simulink model "sampleModel1942"  (R2023a)
settings: Solver=VariableStepAuto  StartTime=0.0  StopTime=10.0  RelTol=1e-3
libraries: hdlsllib x5
settings Model: Creator=user1  LastModifiedBy=user1

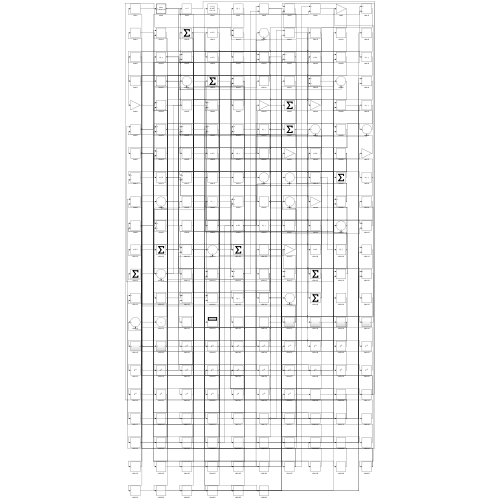
[thumbnail: Simulink's stored preview of the top-level diagram]
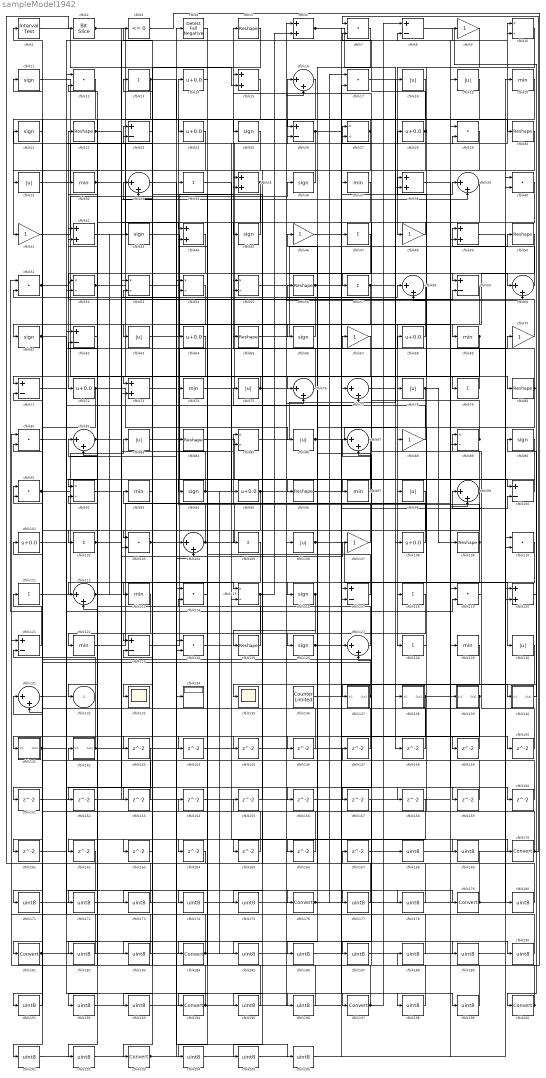
== system sampleModel1942 ==
  cfblk1 : hdlsllib/Logic and Bit Operations/Interval Test  IntervalClosedRight=on  uplimit=0.5  IntervalClosedLeft=on  lowlimit=-0.5  OutDataTypeStr=boolean
  cfblk{10,27,52..55,85,89,92,115} (10 alike) : Product  Inputs=*/  RndMeth=Zero  SaturateOnIntegerOverflow=on
  cfblk{8,23,26,59,62,71,100,117,121,123} (10 alike) : Sum  Inputs=+-
  cfblk{14,24,28,64,68,72,95,101,108} (9 alike) : Bias  Bias=0.0  SaturateOnIntegerOverflow=off
  cfblk{13,34,47,57,79,102,105,111,118,128} (10 alike) : Sum  Inputs=+
  cfblk{7,12,17,29,40,51,81,91,103,110,114,119,124} (13 alike) : DotProduct  OutDataTypeStr=Inherit: Inherit via internal rule
  cfblk{16,33,39,58,60,76..77,82,87,99,104,112,127,131} (14 alike) : Sum  Inputs=|++
  cfblk{18..19,31,63,75,78,83,86,98,106,130} (11 alike) : Abs  SaturateOnIntegerOverflow=off
  cfblk{9,41,46,48,67,70,88,107} (8 alike) : Gain
  cfblk{5,22,30,50,56,65,80,84,96,109,125} (11 alike) : Reshape
  cfblk{11,21,25,36,43,45,61,66,90,94,116,126} (12 alike) : Signum
  cfblk{20,32,37,69,74,93,97,113,122,129} (10 alike) : MinMax
  cfblk{6,15,35,38,42,44,49,73,120} (9 alike) : Sum
  cfblk133 : Scope
  cfblk134 : Display
  cfblk135 : Scope
  cfblk136 : hdlsllib/Sources/Counter Limited  uplimit=7  tsamp=-1
  cfblk137 : Subsystem
      settings: LibrarySourceBlock=|
      | hdlsllib/Ports &
      | Subsystems/Subsystem
  cfblk138 : Subsystem
      settings: LibrarySourceBlock=|
      | hdlsllib/Ports &
      | Subsystems/Subsystem
  cfblk139 : Subsystem
      settings: LibrarySourceBlock=|
      | hdlsllib/Ports &
      | Subsystems/Subsystem
  cfblk140 : Subsystem
      settings: LibrarySourceBlock=|
      | hdlsllib/Ports &
      | Subsystems/Subsystem
  cfblk141 : Subsystem
      settings: LibrarySourceBlock=|
      | hdlsllib/Ports &
      | Subsystems/Subsystem
  cfblk142 : Subsystem
      settings: LibrarySourceBlock=|
      | hdlsllib/Ports &
      | Subsystems/Subsystem
  cfblk{143..167} (25 alike) : Delay  SampleTime=1
  cfblk{168..169,171..175,177..178,180,182..183,185..193,195..196,198..199,201..202,204..206} (30 alike) : DataTypeConversion  OutDataTypeStr=uint8  SaturateOnIntegerOverflow=off  RndMeth=Floor
  cfblk{170,176,179,181,184,194,197,200,203} (9 alike) : DataTypeConversion  SaturateOnIntegerOverflow=off  RndMeth=Floor
  cfblk2 : hdlsllib/Logic and Bit Operations/Bit Slice  lidx=7  ridx=0
  cfblk3 : hdlsllib/Logic and Bit Operations/Compare To Zero  relop=<=  OutDataTypeStr=boolean
  cfblk4 : hdlsllib/Logic and Bit Operations/Detect Fall Negative  vinit=0  OutDataTypeStr=boolean
  cfblk132 : Outport  VectorParamsAs1DForOutWhenUnconnected=off
  wires:
  cfblk111/1 -> cfblk83/1
  cfblk19/1 -> cfblk41/1
  cfblk6/1 -> cfblk108/1, cfblk150/1
  cfblk76/1 -> cfblk5/1
  cfblk126/1 -> cfblk127/1, cfblk169/1
  cfblk2/1 -> cfblk76/1, cfblk30/1
  cfblk124/1 -> cfblk170/1
  cfblk45/1 -> cfblk21/1
  cfblk117/1 -> cfblk93/1
  cfblk78/1 -> cfblk109/1, cfblk146/1
  cfblk15/1 -> cfblk25/1
  cfblk37/1 -> cfblk203/1
  cfblk44/1 -> cfblk72/1
  cfblk43/1 -> cfblk100/1
  cfblk58/1 -> cfblk128/1
  cfblk122/1 -> cfblk85/1
  cfblk114/1 -> cfblk194/1
  cfblk8/1 -> cfblk137/1(In1)
  cfblk33/1 -> cfblk176/1
  cfblk123/1 -> cfblk68/1
  cfblk7/1 -> cfblk126/1
  cfblk66/1 -> cfblk11/1
  cfblk116/1 -> cfblk125/1, cfblk165/1
  cfblk74/1 -> cfblk27/1
  cfblk28/1 -> cfblk116/1, cfblk38/2, cfblk7/2
  cfblk5/1 -> cfblk103/1
  cfblk93/1 -> cfblk23/1
  cfblk42/1 -> cfblk16/1
  cfblk41/1 -> cfblk36/1
  cfblk98/1 -> cfblk113/1
  cfblk138/1(Out1) -> cfblk70/1, cfblk152/1
  cfblk25/1 -> cfblk132/1
  cfblk71/1 -> cfblk67/1
  cfblk115/1 -> cfblk6/2, cfblk193/1
  cfblk139/1(Out1) -> cfblk51/1, cfblk191/1
  cfblk52/1 -> cfblk102/1, cfblk59/2
  cfblk109/1 -> cfblk14/1, cfblk145/1
  cfblk105/1 -> cfblk112/1
  cfblk11/1 -> cfblk99/2
  cfblk99/1 -> cfblk15/1, cfblk175/1
  cfblk107/1 -> cfblk3/1
  cfblk10/1 -> cfblk48/1
  cfblk60/1 -> cfblk49/1
  cfblk84/1 -> cfblk96/1
  cfblk106/1 -> cfblk130/1, cfblk149/1
  cfblk20/1 -> cfblk184/1
  cfblk65/1 -> cfblk19/1
  cfblk85/1 -> cfblk18/1
  cfblk26/1 -> cfblk61/1, cfblk185/1, cfblk190/1
  cfblk86/1 -> cfblk88/1, cfblk39/1, cfblk140/1(In1)
  cfblk61/1 -> cfblk98/1, cfblk159/1, cfblk177/1
  cfblk112/1 -> cfblk107/1, cfblk43/1
  cfblk120/1 -> cfblk200/1
  cfblk36/1 -> cfblk31/1
  cfblk82/1 -> cfblk115/1, cfblk39/2
  cfblk89/1 -> cfblk65/1, cfblk53/2
  cfblk48/1 -> cfblk45/1
  cfblk27/1 -> cfblk24/1, cfblk112/2
  cfblk137/1(Out1) -> cfblk1/1, cfblk71/2
  cfblk21/1 -> cfblk71/1
  cfblk56/1 -> cfblk158/1, cfblk198/1
  cfblk23/1 -> cfblk123/1
  cfblk104/1 -> cfblk74/1, cfblk10/2
  cfblk63/1 -> cfblk35/1
  cfblk140/1(Out1) -> cfblk90/1
  cfblk92/1 -> cfblk85/2
  cfblk70/1 -> cfblk22/1
  cfblk1/1 -> cfblk15/2
  cfblk97/1 -> cfblk56/1
  cfblk17/1 -> cfblk59/1
  cfblk59/1 -> cfblk133/1
  cfblk75/1 -> cfblk55/1, cfblk73/1, cfblk79/1
  cfblk29/1 -> cfblk141/1(In1)
  cfblk127/1 -> cfblk34/1
  cfblk9/1 -> cfblk78/1
  cfblk128/1 -> cfblk38/1
  cfblk100/1 -> cfblk97/1
  cfblk142/1(Out1) -> cfblk17/2, cfblk91/1
  cfblk102/1 -> cfblk9/1, cfblk54/2
  cfblk68/1 -> cfblk66/1
  cfblk4/1 -> cfblk94/1
  cfblk72/1 -> cfblk134/1, cfblk86/1, cfblk201/1
  cfblk55/1 -> cfblk60/1
  cfblk31/1 -> cfblk10/1
  cfblk51/1 -> cfblk52/1, cfblk8/2
  cfblk101/1 -> cfblk28/1
  cfblk39/1 -> cfblk57/1
  cfblk125/1 -> cfblk32/1
  cfblk141/1(Out1) -> cfblk62/1, cfblk77/2, cfblk119/2
  cfblk32/1 -> cfblk44/1, cfblk26/2
  cfblk79/1 -> cfblk27/2
  cfblk69/1 -> cfblk135/1, cfblk127/2
  cfblk88/1 -> cfblk75/1
  cfblk12/1 -> cfblk181/1
  cfblk50/1 -> cfblk69/1
  cfblk113/1 -> cfblk122/1
  cfblk108/1 -> cfblk64/1
  cfblk13/1 -> cfblk63/1, cfblk26/1, cfblk162/1
  cfblk95/1 -> cfblk58/1, cfblk60/2, cfblk161/1
  cfblk46/1 -> cfblk179/1
  cfblk35/1 -> cfblk82/2, cfblk105/1
  cfblk62/1 -> cfblk42/1
  cfblk103/1 -> cfblk50/1, cfblk206/1
  cfblk83/1 -> cfblk115/2
  cfblk136/1 -> cfblk100/2
  cfblk57/1 -> cfblk138/1(In1), cfblk73/2
  cfblk53/1 -> cfblk139/1(In1)
  cfblk80/1 -> cfblk118/1, cfblk55/2
  cfblk121/1 -> cfblk111/1
  cfblk91/1 -> cfblk4/1, cfblk196/1
  cfblk67/1 -> cfblk92/1
  cfblk22/1 -> cfblk80/1, cfblk156/1
  cfblk94/1 -> cfblk29/2, cfblk84/1
  cfblk81/1 -> cfblk197/1
  cfblk119/1 -> cfblk89/1
  cfblk18/1 -> cfblk143/1
  cfblk14/1 -> cfblk144/1
  cfblk145/1 -> cfblk16/2
  cfblk146/1 -> cfblk53/1
  cfblk147/1 -> cfblk23/2
  cfblk77/1 -> cfblk148/1
  cfblk148/1 -> cfblk82/1
  cfblk149/1 -> cfblk54/1
  cfblk150/1 -> cfblk99/1
  cfblk64/1 -> cfblk151/1
  cfblk151/1 -> cfblk76/2
  cfblk152/1 -> cfblk103/2
  cfblk118/1 -> cfblk153/1
  cfblk153/1 -> cfblk62/2
  cfblk154/1 -> cfblk29/1
  cfblk155/1 -> cfblk35/2
  cfblk156/1 -> cfblk89/2
  cfblk110/1 -> cfblk157/1
  cfblk159/1 -> cfblk44/2
  cfblk38/1 -> cfblk160/1
  cfblk160/1 -> cfblk51/2
  cfblk161/1 -> cfblk52/2
  cfblk24/1 -> cfblk163/1
  cfblk163/1 -> cfblk123/2
  cfblk90/1 -> cfblk164/1
  cfblk164/1 -> cfblk2/1
  cfblk165/1 -> cfblk91/2
  cfblk34/1 -> cfblk166/1
  cfblk166/1 -> cfblk42/2
  cfblk167/1 -> cfblk168/1
  cfblk168/1 -> cfblk7/1
  cfblk169/1 -> cfblk167/1
  cfblk170/1 -> cfblk58/2, cfblk101/1
  cfblk54/1 -> cfblk171/1
  cfblk171/1 -> cfblk124/1
  cfblk162/1 -> cfblk172/1
  cfblk172/1 -> cfblk124/2
  cfblk40/1 -> cfblk173/1
  cfblk173/1 -> cfblk142/1(In1)
  cfblk144/1 -> cfblk174/1
  cfblk174/1 -> cfblk40/1
  cfblk175/1 -> cfblk40/2
  cfblk176/1 -> cfblk49/2, cfblk17/1
  cfblk177/1 -> cfblk33/1
  cfblk96/1 -> cfblk178/1
  cfblk178/1 -> cfblk33/2
  cfblk179/1 -> cfblk155/1, cfblk154/1
  cfblk49/1 -> cfblk180/1
  cfblk180/1 -> cfblk46/1
  cfblk181/1 -> cfblk104/2, cfblk119/1
  cfblk143/1 -> cfblk182/1
  cfblk182/1 -> cfblk12/1
  cfblk16/1 -> cfblk183/1
  cfblk183/1 -> cfblk12/2
  cfblk184/1 -> cfblk121/1, cfblk95/1
  cfblk185/1 -> cfblk20/1
  cfblk87/1 -> cfblk186/1
  cfblk186/1 -> cfblk110/1
  cfblk157/1 -> cfblk187/1
  cfblk187/1 -> cfblk87/1
  cfblk3/1 -> cfblk188/1
  cfblk188/1 -> cfblk87/2
  cfblk131/1 -> cfblk189/1
  cfblk189/1 -> cfblk110/2
  cfblk190/1 -> cfblk131/1
  cfblk191/1 -> cfblk131/2
  cfblk47/1 -> cfblk192/1
  cfblk192/1 -> cfblk106/1
  cfblk193/1 -> cfblk47/1
  cfblk194/1 -> cfblk92/2, cfblk77/1
  cfblk130/1 -> cfblk195/1
  cfblk195/1 -> cfblk114/1
  cfblk196/1 -> cfblk114/2
  cfblk197/1 -> cfblk121/2, cfblk6/1, cfblk8/1
  cfblk198/1 -> cfblk81/1
  cfblk73/1 -> cfblk199/1
  cfblk199/1 -> cfblk81/2
  cfblk200/1 -> cfblk147/1, cfblk13/1
  cfblk201/1 -> cfblk120/1
  cfblk158/1 -> cfblk202/1
  cfblk202/1 -> cfblk120/2
  cfblk203/1 -> cfblk104/1, cfblk117/1
  cfblk30/1 -> cfblk204/1
  cfblk204/1 -> cfblk37/1
  cfblk129/1 -> cfblk205/1
  cfblk205/1 -> cfblk117/2
  cfblk206/1 -> cfblk129/1

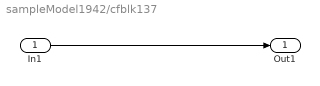
== system sampleModel1942/cfblk137 ==
  In1 : Inport
  Out1 : Outport
  wires:
  In1/1 -> Out1/1

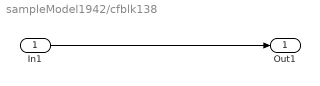
== system sampleModel1942/cfblk138 ==
  In1 : Inport
  Out1 : Outport
  wires:
  In1/1 -> Out1/1

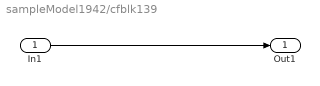
== system sampleModel1942/cfblk139 ==
  In1 : Inport
  Out1 : Outport
  wires:
  In1/1 -> Out1/1

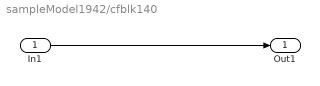
== system sampleModel1942/cfblk140 ==
  In1 : Inport
  Out1 : Outport
  wires:
  In1/1 -> Out1/1

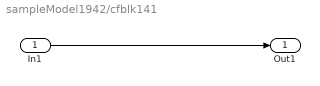
== system sampleModel1942/cfblk141 ==
  In1 : Inport
  Out1 : Outport
  wires:
  In1/1 -> Out1/1

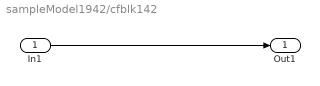
== system sampleModel1942/cfblk142 ==
  In1 : Inport
  Out1 : Outport
  wires:
  In1/1 -> Out1/1
